simulink model "wbs_sim"  (R2025a)
settings: Solver=FixedStepAuto  StartTime=0.0  StopTime=20  FixedStep=0.001  RelTol=1e-3
undefined symbols (not defined in the file): dyaw, L_l, L_r, phi_1l, phi_1r, phi_4l, phi_4r, roll, theta_l, theta_r, x, X, Y, yaw, Z
libraries: sm_lib x86, nesl_utility x28, slpidlib x6
(part 3 of 4)

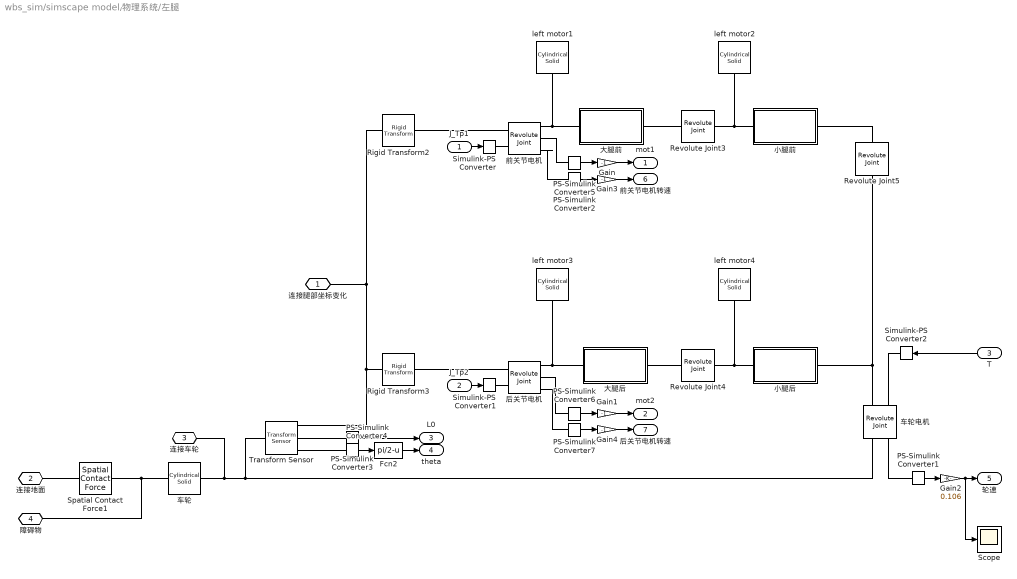
== system wbs_sim/simscape model/物理系统/左腿 ==
  J_Tp1 : Inport
  J_Tp2 : Inport  Port=2
  T : Inport  Port=3
  Fcn2 : Fcn  Expr=pi/2-u
  Gain{,1,3..4} (4 alike) : Gain  Gain=-1
  Gain2 : Gain  Gain=0.106
  PS-Simulink Converter{1..7} (7 alike) : nesl_utility/PS-Simulink Converter  PhysicalDomain=network_engine_domain  SubClassName=ps_output  LeftPortType=input  RightPortType=output  PseudoPeriodic=off  Frequencies=[]  VectorFormat=inherit  Unit=inherit  AffineConversion=off
  Revolute Joint3 : sm_lib/Joints/Revolute Joint  JointMode=Normal  CompositeWrenchDir=FollowerOnBase  CompositeWrenchFrame=BaseFrame  SenseConstraintForce=off  SenseConstraintTorque=off  SenseTotalForce=off  SenseTotalTorque=off  PositionTargetSpecify=on  PositionTargetPriority=Low  PositionTargetValue=-135  PositionTargetValueUnits=deg  VelocityTargetSpecify=off  VelocityTargetPriority=High  VelocityTargetValue=90  VelocityTargetValueUnits=deg/s  EquilibriumPosition=0  EquilibriumPositionUnits=deg  SpringStiffness=0  SpringStiffnessUnits=N*m/deg  DampingCoefficient=0  DampingCoefficientUnits=N*m/(deg/s)  LowerLimitSpecify=off  LowerLimitBound=-90  LowerLimitBoundUnits=deg  LowerLimitStiffness=1e4  LowerLimitStiffnessUnits=N*m/deg  LowerLimitDamping=10  LowerLimitDampingUnits=N*m/(deg/s)  LowerLimitTransitionRegionWidth=0.1  LowerLimitTransitionRegionWidthUnits=deg  UpperLimitSpecify=off  UpperLimitBound=90  UpperLimitBoundUnits=deg  UpperLimitStiffness=1e4  UpperLimitStiffnessUnits=N*m/deg  UpperLimitDamping=10  UpperLimitDampingUnits=N*m/(deg/s)  UpperLimitTransitionRegionWidth=0.1  UpperLimitTransitionRegionWidthUnits=deg  TorqueActuationMode=NoTorque  MotionActuationMode=ComputedMotion  SensePosition=off  SenseVelocity=off  SenseAcceleration=off  SenseTorqueForce=off  SenseLowerLimitTorqueForce=off  SenseUpperLimitTorqueForce=off
  Revolute Joint4 : sm_lib/Joints/Revolute Joint  JointMode=Normal  CompositeWrenchDir=FollowerOnBase  CompositeWrenchFrame=BaseFrame  SenseConstraintForce=off  SenseConstraintTorque=off  SenseTotalForce=off  SenseTotalTorque=off  PositionTargetSpecify=off  PositionTargetPriority=High  PositionTargetValue=0  PositionTargetValueUnits=deg  VelocityTargetSpecify=off  VelocityTargetPriority=High  VelocityTargetValue=90  VelocityTargetValueUnits=deg/s  EquilibriumPosition=0  EquilibriumPositionUnits=deg  SpringStiffness=0  SpringStiffnessUnits=N*m/deg  DampingCoefficient=0  DampingCoefficientUnits=N*m/(deg/s)  LowerLimitSpecify=off  LowerLimitBound=-90  LowerLimitBoundUnits=deg  LowerLimitStiffness=1e4  LowerLimitStiffnessUnits=N*m/deg  LowerLimitDamping=10  LowerLimitDampingUnits=N*m/(deg/s)  LowerLimitTransitionRegionWidth=0.1  LowerLimitTransitionRegionWidthUnits=deg  UpperLimitSpecify=off  UpperLimitBound=90  UpperLimitBoundUnits=deg  UpperLimitStiffness=1e4  UpperLimitStiffnessUnits=N*m/deg  UpperLimitDamping=10  UpperLimitDampingUnits=N*m/(deg/s)  UpperLimitTransitionRegionWidth=0.1  UpperLimitTransitionRegionWidthUnits=deg  TorqueActuationMode=NoTorque  MotionActuationMode=ComputedMotion  SensePosition=off  SenseVelocity=off  SenseAcceleration=off  SenseTorqueForce=off  SenseLowerLimitTorqueForce=off  SenseUpperLimitTorqueForce=off
  Revolute Joint5 : sm_lib/Joints/Revolute Joint  JointMode=Normal  CompositeWrenchDir=FollowerOnBase  CompositeWrenchFrame=BaseFrame  SenseConstraintForce=off  SenseConstraintTorque=off  SenseTotalForce=off  SenseTotalTorque=off  PositionTargetSpecify=off  PositionTargetPriority=High  PositionTargetValue=0  PositionTargetValueUnits=deg  VelocityTargetSpecify=off  VelocityTargetPriority=High  VelocityTargetValue=90  VelocityTargetValueUnits=deg/s  EquilibriumPosition=0  EquilibriumPositionUnits=deg  SpringStiffness=0  SpringStiffnessUnits=N*m/deg  DampingCoefficient=0  DampingCoefficientUnits=N*m/(deg/s)  LowerLimitSpecify=off  LowerLimitBound=-90  LowerLimitBoundUnits=deg  LowerLimitStiffness=1e4  LowerLimitStiffnessUnits=N*m/deg  LowerLimitDamping=10  LowerLimitDampingUnits=N*m/(deg/s)  LowerLimitTransitionRegionWidth=0.1  LowerLimitTransitionRegionWidthUnits=deg  UpperLimitSpecify=off  UpperLimitBound=90  UpperLimitBoundUnits=deg  UpperLimitStiffness=1e4  UpperLimitStiffnessUnits=N*m/deg  UpperLimitDamping=10  UpperLimitDampingUnits=N*m/(deg/s)  UpperLimitTransitionRegionWidth=0.1  UpperLimitTransitionRegionWidthUnits=deg  TorqueActuationMode=NoTorque  MotionActuationMode=ComputedMotion  SensePosition=off  SenseVelocity=off  SenseAcceleration=off  SenseTorqueForce=off  SenseLowerLimitTorqueForce=off  SenseUpperLimitTorqueForce=off
  Rigid Transform2 : sm_lib/Frames and Transforms/Rigid Transform  RotationMethod=None  FollAlignAxisA=+X  BaseAlignAxisA=+Y  FollAlignAxisB=+Y  BaseAlignAxisB=+Z  RotationStandardAxis=+Z  RotationAngle=0.0  RotationAngleUnits=deg  RotationArbitraryAxis=[0 0 1]  RotationSequenceAxes=FollowerAxes  RotationSequence=XYX  RotationSequenceAngles=[0 0 0]  RotationSequenceAnglesUnits=deg  RotationMatrix=[1 0 0; 0 1 0; 0 0 1]  Quaternion=[1 0 0 0]  TranslationMethod=StandardAxis  TranslationCartesianOffset=[0 0 0]  TranslationCartesianOffsetUnits=m  TranslationStandardAxis=+X  TranslationStandardOffset=0.0425  TranslationStandardOffsetUnits=m  TranslationROffset=0  TranslationROffsetUnits=m  TranslationThetaOffset=0  TranslationThetaOffsetUnits=deg  TranslationZOffset=0  TranslationZOffsetUnits=m
  Rigid Transform3 : sm_lib/Frames and Transforms/Rigid Transform  RotationMethod=None  FollAlignAxisA=+X  BaseAlignAxisA=+Y  FollAlignAxisB=+Y  BaseAlignAxisB=+Z  RotationStandardAxis=+Z  RotationAngle=0.0  RotationAngleUnits=deg  RotationArbitraryAxis=[0 0 1]  RotationSequenceAxes=FollowerAxes  RotationSequence=XYX  RotationSequenceAngles=[0 0 0]  RotationSequenceAnglesUnits=deg  RotationMatrix=[1 0 0; 0 1 0; 0 0 1]  Quaternion=[1 0 0 0]  TranslationMethod=StandardAxis  TranslationCartesianOffset=[0 0 0]  TranslationCartesianOffsetUnits=m  TranslationStandardAxis=-X  TranslationStandardOffset=0.0425  TranslationStandardOffsetUnits=m  TranslationROffset=0  TranslationROffsetUnits=m  TranslationThetaOffset=0  TranslationThetaOffsetUnits=deg  TranslationZOffset=0  TranslationZOffsetUnits=m
  Scope : Scope
      settings: ActiveDisplayYMinimum=-32.212491116980587  ActiveDisplayYMaximum=60.605287499899276  DataLoggingVariableName=ScopeData7
  Simulink-PS Converter : nesl_utility/Simulink-PS Converter  PhysicalDomain=network_engine_domain  SubClassName=ps_input  LeftPortType=input  RightPortType=output  PseudoPeriodic=off  Frequencies=[]  NoiseDistribution=none  NoiseParameters=[]  Unit=1  AffineConversion=off  FilteringAndDerivatives=provide  SimscapeFilterOrder=1  InputFilterTimeConstant=0.001  UdotUserProvided=0
  Simulink-PS Converter1 : nesl_utility/Simulink-PS Converter  PhysicalDomain=network_engine_domain  SubClassName=ps_input  LeftPortType=input  RightPortType=output  PseudoPeriodic=off  Frequencies=[]  NoiseDistribution=none  NoiseParameters=[]  Unit=1  AffineConversion=off  FilteringAndDerivatives=provide  SimscapeFilterOrder=1  InputFilterTimeConstant=0.001  UdotUserProvided=0
  Simulink-PS Converter2 : nesl_utility/Simulink-PS Converter  PhysicalDomain=network_engine_domain  SubClassName=ps_input  LeftPortType=input  RightPortType=output  PseudoPeriodic=off  Frequencies=[]  NoiseDistribution=none  NoiseParameters=[]  Unit=1  AffineConversion=off  FilteringAndDerivatives=provide  SimscapeFilterOrder=1  InputFilterTimeConstant=0.001  UdotUserProvided=0
  Spatial Contact Force1 : sm_lib/Forces and Torques/Spatial Contact Force  SenseSeparationDistance=off  NormalForceType=SmoothSpringDamper  NormalStiffness=1e6  NormalStiffnessUnits=N/m  NormalDamping=1e3  NormalDampingUnits=N/(m/s)  NormalTransitionRegionWidth=1e-4  NormalTransitionRegionWidthUnits=m  FrictionType=SmoothStickSlip  CoefficientOfStaticFriction=0.5  CoefficientOfDynamicFriction=0.3  FrictionalCriticalVelocity=1e-3  FrictionalCriticalVelocityUnits=m/s  SenseContactSignal=off  SensePenetrationDepth=off  SenseNormalVelocity=off  SenseTangentialVelocity=off  SensingForceTorqueDirection=BaseOnFollower  SensingForceTorqueResolutionFrame=ContactFrame  SenseNormalForce=off  SenseNormalForceMagnitude=off  SenseNormalTorque=off  SenseFrictionalForce=off  SenseFrictionalForceMagnitude=off  SenseFrictionalTorque=off  SenseTotalForce=off  SenseTotalTorque=off  SenseContactBaseRotation=off  SenseContactBaseTranslation=off  SenseContactFollowerRotation=off  SenseContactFollowerTranslation=off  ZeroCrossDetectContactStartAndEnd=off
  Transform Sensor : sm_lib/Frames and Transforms/Transform Sensor  MeasurementFrame=World  RotationSequence=XYX  SenseAngle=off  SenseAxis=off  SenseQ=off  SenseR=off  SenseRotationSequence=off  SenseOmegaX=off  SenseOmegaY=off  SenseOmegaZ=off  SenseOmega=off  SenseQDot=off  SenseRDot=off  SenseRotationSequenceDot=off  SenseAlphaX=off  SenseAlphaY=off  SenseAlphaZ=off  SenseAlpha=off  SenseQDDot=off  SenseRDDot=off  SenseX=off  SenseY=off  SenseZ=off  SenseXYZ=off  SenseRad=on  SenseAzim=on  SenseDist=off  SenseInc=off  SenseXDot=off  SenseYDot=off  SenseZDot=off  SenseXYZDot=off  SenseRadDot=off  SenseAzimDot=off  SenseDistDot=off  SenseIncDot=off  SenseXDDot=off  SenseYDDot=off  SenseZDDot=off  SenseXYZDDot=off  SenseRadDDot=off  SenseAzimDDot=off  SenseDistDDot=off  SenseIncDDot=off
  left motor{1..4} (4 alike) : sm_lib/Body Elements/Cylindrical Solid  CylinderRadius=0.03  CylinderRadiusUnits=m  CylinderLength=0.02  CylinderLengthUnits=m  ExportEntireGeometry=off  InertiaType=CalculateFromGeometry  BasedOnType=Mass  Density=1000  DensityUnits=kg/m^3  Mass=0  MassUnits=kg  CenterOfMass=[0 0 0]  CenterOfMassUnits=m  MomentsOfInertia=[1 1 1]  MomentsOfInertiaUnits=kg*m^2  ProductsOfInertia=[0 0 0]  ProductsOfInertiaUnits=kg*m^2  GraphicType=FromGeometry  MarkerShape=Sphere  MarkerSize=10  GraphicVisPropType=SimpleVisualProperties  GraphicDiffuseColor=[0.1569 0.1569 0.03137]  GraphicOpacity=1.0  GraphicSpecularColor=[0.5 0.5 0.5 1.0]  GraphicAmbientColor=[0.15 0.15 0.15 1.0]  GraphicEmissiveColor=[0.0 0.0 0.0 1.0]  GraphicShininess=75  DoExposeReferenceFrame=on  SerializedFrames=<Frames/>
  前关节电机 : sm_lib/Joints/Revolute Joint  JointMode=Normal  CompositeWrenchDir=FollowerOnBase  CompositeWrenchFrame=BaseFrame  SenseConstraintForce=off  SenseConstraintTorque=off  SenseTotalForce=off  SenseTotalTorque=off  PositionTargetSpecify=on  PositionTargetPriority=High  PositionTargetValue=-30  PositionTargetValueUnits=deg  VelocityTargetSpecify=off  VelocityTargetPriority=High  VelocityTargetValue=90  VelocityTargetValueUnits=deg/s  EquilibriumPosition=0  EquilibriumPositionUnits=deg  SpringStiffness=0  SpringStiffnessUnits=N*m/deg  DampingCoefficient=0  DampingCoefficientUnits=N*m/(deg/s)  LowerLimitSpecify=off  LowerLimitBound=-90  LowerLimitBoundUnits=deg  LowerLimitStiffness=1e4  LowerLimitStiffnessUnits=N*m/deg  LowerLimitDamping=10  LowerLimitDampingUnits=N*m/(deg/s)  LowerLimitTransitionRegionWidth=0.1  LowerLimitTransitionRegionWidthUnits=deg  UpperLimitSpecify=off  UpperLimitBound=90  UpperLimitBoundUnits=deg  UpperLimitStiffness=1e4  UpperLimitStiffnessUnits=N*m/deg  UpperLimitDamping=10  UpperLimitDampingUnits=N*m/(deg/s)  UpperLimitTransitionRegionWidth=0.1  UpperLimitTransitionRegionWidthUnits=deg  TorqueActuationMode=InputTorque  MotionActuationMode=ComputedMotion  SensePosition=on  SenseVelocity=on  SenseAcceleration=off  SenseTorqueForce=off  SenseLowerLimitTorqueForce=off  SenseUpperLimitTorqueForce=off
  后关节电机 : sm_lib/Joints/Revolute Joint  JointMode=Normal  CompositeWrenchDir=FollowerOnBase  CompositeWrenchFrame=BaseFrame  SenseConstraintForce=off  SenseConstraintTorque=off  SenseTotalForce=off  SenseTotalTorque=off  PositionTargetSpecify=on  PositionTargetPriority=High  PositionTargetValue=210  PositionTargetValueUnits=deg  VelocityTargetSpecify=off  VelocityTargetPriority=High  VelocityTargetValue=90  VelocityTargetValueUnits=deg/s  EquilibriumPosition=0  EquilibriumPositionUnits=deg  SpringStiffness=0  SpringStiffnessUnits=N*m/deg  DampingCoefficient=0  DampingCoefficientUnits=N*m/(deg/s)  LowerLimitSpecify=off  LowerLimitBound=-90  LowerLimitBoundUnits=deg  LowerLimitStiffness=1e4  LowerLimitStiffnessUnits=N*m/deg  LowerLimitDamping=10  LowerLimitDampingUnits=N*m/(deg/s)  LowerLimitTransitionRegionWidth=0.1  LowerLimitTransitionRegionWidthUnits=deg  UpperLimitSpecify=off  UpperLimitBound=90  UpperLimitBoundUnits=deg  UpperLimitStiffness=1e4  UpperLimitStiffnessUnits=N*m/deg  UpperLimitDamping=10  UpperLimitDampingUnits=N*m/(deg/s)  UpperLimitTransitionRegionWidth=0.1  UpperLimitTransitionRegionWidthUnits=deg  TorqueActuationMode=InputTorque  MotionActuationMode=ComputedMotion  SensePosition=on  SenseVelocity=on  SenseAcceleration=off  SenseTorqueForce=off  SenseLowerLimitTorqueForce=off  SenseUpperLimitTorqueForce=off
  大腿前 : Subsystem  mask{L=0.21, W=0.01, H=0.05, mass=0.75}
      mask prompts: L "Length"; W "Width"; H "Height"
  大腿后 : Subsystem  mask{L=0.21, W=0.01, H=0.05, mass=0.75}
      mask prompts: L "Length"; W "Width"; H "Height"
  小腿前 : Subsystem  mask{L=0.25, W=0.01, H=0.05, mass=0.5}
      mask prompts: L "Length"; W "Width"; H "Height"
  小腿后 : Subsystem  mask{L=0.25, W=0.01, H=0.05, mass=0.5}
      mask prompts: L "Length"; W "Width"; H "Height"
  车轮 : sm_lib/Body Elements/Cylindrical Solid  CylinderRadius=0.06  CylinderRadiusUnits=m  CylinderLength=0.03  CylinderLengthUnits=m  ExportEntireGeometry=on  InertiaType=CalculateFromGeometry  BasedOnType=Mass  Density=661  DensityUnits=kg/m^3  Mass=0.5  MassUnits=kg  CenterOfMass=[0 0 0]  CenterOfMassUnits=m  MomentsOfInertia=[1 1 1]  MomentsOfInertiaUnits=kg*m^2  ProductsOfInertia=[0 0 0]  ProductsOfInertiaUnits=kg*m^2  GraphicType=FromGeometry  MarkerShape=Sphere  MarkerSize=10  GraphicVisPropType=SimpleVisualProperties  GraphicDiffuseColor=[1 0 0]  GraphicOpacity=1.0  GraphicSpecularColor=[0.5 0.5 0.5 1.0]  GraphicAmbientColor=[0.15 0.15 0.15 1.0]  GraphicEmissiveColor=[0.0 0.0 0.0 1.0]  GraphicShininess=75  DoExposeReferenceFrame=on  SerializedFrames=<Frames/>
  车轮电机 : sm_lib/Joints/Revolute Joint  JointMode=Normal  CompositeWrenchDir=FollowerOnBase  CompositeWrenchFrame=BaseFrame  SenseConstraintForce=off  SenseConstraintTorque=off  SenseTotalForce=off  SenseTotalTorque=off  PositionTargetSpecify=off  PositionTargetPriority=High  PositionTargetValue=0  PositionTargetValueUnits=deg  VelocityTargetSpecify=off  VelocityTargetPriority=High  VelocityTargetValue=90  VelocityTargetValueUnits=deg/s  EquilibriumPosition=0  EquilibriumPositionUnits=deg  SpringStiffness=0  SpringStiffnessUnits=N*m/deg  DampingCoefficient=0  DampingCoefficientUnits=N*m/(deg/s)  LowerLimitSpecify=off  LowerLimitBound=-90  LowerLimitBoundUnits=deg  LowerLimitStiffness=1e4  LowerLimitStiffnessUnits=N*m/deg  LowerLimitDamping=10  LowerLimitDampingUnits=N*m/(deg/s)  LowerLimitTransitionRegionWidth=0.1  LowerLimitTransitionRegionWidthUnits=deg  UpperLimitSpecify=off  UpperLimitBound=90  UpperLimitBoundUnits=deg  UpperLimitStiffness=1e4  UpperLimitStiffnessUnits=N*m/deg  UpperLimitDamping=10  UpperLimitDampingUnits=N*m/(deg/s)  UpperLimitTransitionRegionWidth=0.1  UpperLimitTransitionRegionWidthUnits=deg  TorqueActuationMode=InputTorque  MotionActuationMode=ComputedMotion  SensePosition=off  SenseVelocity=on  SenseAcceleration=off  SenseTorqueForce=off  SenseLowerLimitTorqueForce=off  SenseUpperLimitTorqueForce=off
  连接腿部坐标变化 : PMIOPort  Side=Left
  连接地面 : PMIOPort  Port=2  Side=Left
  连接车轮 : PMIOPort  Port=3  Side=Left
  障碍物 : PMIOPort  Port=4  Side=Left
  mot1 : Outport
  mot2 : Outport  Port=2
  L0 : Outport  Port=3
  theta : Outport  Port=4
  轮速 : Outport  Port=5
  前关节电机转速 : Outport  Port=6
  后关节电机转速 : Outport  Port=7
  wires:
  T/1 -> Simulink-PS Converter2/1
  J_Tp2/1 -> Simulink-PS Converter1/1
  J_Tp1/1 -> Simulink-PS Converter/1
  Gain/1 -> mot1/1
  PS-Simulink Converter5/1 -> Gain/1
  Gain1/1 -> mot2/1
  PS-Simulink Converter6/1 -> Gain1/1
  PS-Simulink Converter3/1 -> L0/1
  Fcn2/1 -> theta/1
  PS-Simulink Converter4/1 -> Fcn2/1
  Gain2/1 -> Scope/1, 轮速/1
  PS-Simulink Converter1/1 -> Gain2/1
  PS-Simulink Converter2/1 -> Gain3/1
  Gain3/1 -> 前关节电机转速/1
  Gain4/1 -> 后关节电机转速/1
  PS-Simulink Converter7/1 -> Gain4/1
  connections:
  前关节电机/LConn1 -- Rigid Transform2/RConn1
  Simulink-PS Converter1/RConn1 -- 后关节电机/LConn2
  Simulink-PS Converter2/RConn1 -- 车轮电机/LConn2
  Rigid Transform2/LConn1 -- Transform Sensor/RConn1 -- Rigid Transform3/LConn1 -- 连接腿部坐标变化/RConn1
  车轮电机/LConn1 -- 小腿后/RConn1 -- Revolute Joint5/LConn1
  Revolute Joint4/LConn1 -- 大腿后/RConn1
  车轮/LConn1 -- 障碍物/RConn1 -- Spatial Contact Force1/RConn1
  大腿后/LConn1 -- left motor3/RConn1 -- 后关节电机/RConn1
  后关节电机/LConn1 -- Rigid Transform3/RConn1
  Simulink-PS Converter/RConn1 -- 前关节电机/LConn2
  大腿前/LConn1 -- left motor1/RConn1 -- 前关节电机/RConn1
  Revolute Joint3/LConn1 -- 大腿前/RConn1
  小腿后/LConn1 -- left motor4/RConn1 -- Revolute Joint4/RConn1
  Revolute Joint3/RConn1 -- left motor2/RConn1 -- 小腿前/LConn1
  车轮/RConn1 -- 车轮电机/RConn1 -- Transform Sensor/LConn1 -- 连接车轮/RConn1
  小腿前/RConn1 -- Revolute Joint5/RConn1
  Spatial Contact Force1/LConn1 -- 连接地面/RConn1
  PS-Simulink Converter5/LConn1 -- 前关节电机/RConn2
  后关节电机/RConn2 -- PS-Simulink Converter6/LConn1
  PS-Simulink Converter3/LConn1 -- Transform Sensor/RConn2
  Transform Sensor/RConn3 -- PS-Simulink Converter4/LConn1
  PS-Simulink Converter1/LConn1 -- 车轮电机/RConn2
  前关节电机/RConn3 -- PS-Simulink Converter2/LConn1
  后关节电机/RConn3 -- PS-Simulink Converter7/LConn1

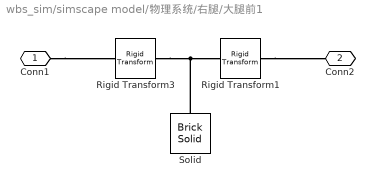
== system wbs_sim/simscape model/物理系统/右腿/大腿前1 ==
  Rigid Transform1 : sm_lib/Frames and Transforms/Rigid Transform  RotationMethod=None  FollAlignAxisA=+X  BaseAlignAxisA=+Y  FollAlignAxisB=+Y  BaseAlignAxisB=+Z  RotationStandardAxis=+Z  RotationAngle=0.0  RotationAngleUnits=deg  RotationArbitraryAxis=[0 0 1]  RotationSequenceAxes=FollowerAxes  RotationSequence=XYX  RotationSequenceAngles=[0 0 0]  RotationSequenceAnglesUnits=deg  RotationMatrix=[1 0 0; 0 1 0; 0 0 1]  Quaternion=[1 0 0 0]  TranslationMethod=StandardAxis  TranslationCartesianOffset=[0 0 0]  TranslationCartesianOffsetUnits=m  TranslationStandardAxis=+X  TranslationStandardOffset=L/2  TranslationStandardOffsetUnits=m  TranslationROffset=0  TranslationROffsetUnits=m  TranslationThetaOffset=0  TranslationThetaOffsetUnits=deg  TranslationZOffset=0  TranslationZOffsetUnits=m
  Rigid Transform3 : sm_lib/Frames and Transforms/Rigid Transform  RotationMethod=None  FollAlignAxisA=+X  BaseAlignAxisA=+Y  FollAlignAxisB=+Y  BaseAlignAxisB=+Z  RotationStandardAxis=+Z  RotationAngle=0.0  RotationAngleUnits=deg  RotationArbitraryAxis=[0 0 1]  RotationSequenceAxes=FollowerAxes  RotationSequence=XYX  RotationSequenceAngles=[0 0 0]  RotationSequenceAnglesUnits=deg  RotationMatrix=[1 0 0; 0 1 0; 0 0 1]  Quaternion=[1 0 0 0]  TranslationMethod=StandardAxis  TranslationCartesianOffset=[0 0 0]  TranslationCartesianOffsetUnits=m  TranslationStandardAxis=+X  TranslationStandardOffset=L/2  TranslationStandardOffsetUnits=m  TranslationROffset=0  TranslationROffsetUnits=m  TranslationThetaOffset=0  TranslationThetaOffsetUnits=deg  TranslationZOffset=0  TranslationZOffsetUnits=m
  Solid : sm_lib/Body Elements/Brick Solid  BrickDimensions=[L H W]  BrickDimensionsUnits=m  ExportEntireGeometry=off  InertiaType=CalculateFromGeometry  BasedOnType=Mass  Density=Mass  DensityUnits=kg/m^3  Mass=mass  MassUnits=kg  CenterOfMass=[0 0 0]  CenterOfMassUnits=m  MomentsOfInertia=[1 1 1]  MomentsOfInertiaUnits=kg*m^2  ProductsOfInertia=[0 0 0]  ProductsOfInertiaUnits=kg*m^2  GraphicType=FromGeometry  MarkerShape=Sphere  MarkerSize=10  GraphicVisPropType=SimpleVisualProperties  GraphicDiffuseColor=[0.6667 0 1]  GraphicOpacity=1.0  GraphicSpecularColor=[0.5 0.5 0.5 1.0]  GraphicAmbientColor=[0.15 0.15 0.15 1.0]  GraphicEmissiveColor=[0.0 0.0 0.0 1.0]  GraphicShininess=75  DoExposeReferenceFrame=on  SerializedFrames=<Frames/>
  Conn1 : PMIOPort  Side=Left
  Conn2 : PMIOPort  Port=2  Side=Right
  connections:
  Solid/RConn1 -- Rigid Transform3/RConn1 -- Rigid Transform1/LConn1
  Conn1/RConn1 -- Rigid Transform3/LConn1
  Rigid Transform1/RConn1 -- Conn2/RConn1

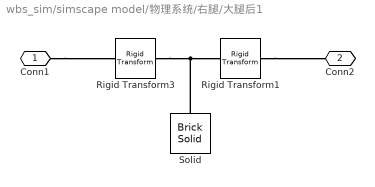
== system wbs_sim/simscape model/物理系统/右腿/大腿后1 ==
  Rigid Transform1 : sm_lib/Frames and Transforms/Rigid Transform  RotationMethod=None  FollAlignAxisA=+X  BaseAlignAxisA=+Y  FollAlignAxisB=+Y  BaseAlignAxisB=+Z  RotationStandardAxis=+Z  RotationAngle=0.0  RotationAngleUnits=deg  RotationArbitraryAxis=[0 0 1]  RotationSequenceAxes=FollowerAxes  RotationSequence=XYX  RotationSequenceAngles=[0 0 0]  RotationSequenceAnglesUnits=deg  RotationMatrix=[1 0 0; 0 1 0; 0 0 1]  Quaternion=[1 0 0 0]  TranslationMethod=StandardAxis  TranslationCartesianOffset=[0 0 0]  TranslationCartesianOffsetUnits=m  TranslationStandardAxis=+X  TranslationStandardOffset=L/2  TranslationStandardOffsetUnits=m  TranslationROffset=0  TranslationROffsetUnits=m  TranslationThetaOffset=0  TranslationThetaOffsetUnits=deg  TranslationZOffset=0  TranslationZOffsetUnits=m
  Rigid Transform3 : sm_lib/Frames and Transforms/Rigid Transform  RotationMethod=None  FollAlignAxisA=+X  BaseAlignAxisA=+Y  FollAlignAxisB=+Y  BaseAlignAxisB=+Z  RotationStandardAxis=+Z  RotationAngle=0.0  RotationAngleUnits=deg  RotationArbitraryAxis=[0 0 1]  RotationSequenceAxes=FollowerAxes  RotationSequence=XYX  RotationSequenceAngles=[0 0 0]  RotationSequenceAnglesUnits=deg  RotationMatrix=[1 0 0; 0 1 0; 0 0 1]  Quaternion=[1 0 0 0]  TranslationMethod=StandardAxis  TranslationCartesianOffset=[0 0 0]  TranslationCartesianOffsetUnits=m  TranslationStandardAxis=+X  TranslationStandardOffset=L/2  TranslationStandardOffsetUnits=m  TranslationROffset=0  TranslationROffsetUnits=m  TranslationThetaOffset=0  TranslationThetaOffsetUnits=deg  TranslationZOffset=0  TranslationZOffsetUnits=m
  Solid : sm_lib/Body Elements/Brick Solid  BrickDimensions=[L H W]  BrickDimensionsUnits=m  ExportEntireGeometry=off  InertiaType=CalculateFromGeometry  BasedOnType=Mass  Density=Mass  DensityUnits=kg/m^3  Mass=mass  MassUnits=kg  CenterOfMass=[0 0 0]  CenterOfMassUnits=m  MomentsOfInertia=[1 1 1]  MomentsOfInertiaUnits=kg*m^2  ProductsOfInertia=[0 0 0]  ProductsOfInertiaUnits=kg*m^2  GraphicType=FromGeometry  MarkerShape=Sphere  MarkerSize=10  GraphicVisPropType=SimpleVisualProperties  GraphicDiffuseColor=[0.6667 0 1]  GraphicOpacity=1.0  GraphicSpecularColor=[0.5 0.5 0.5 1.0]  GraphicAmbientColor=[0.15 0.15 0.15 1.0]  GraphicEmissiveColor=[0.0 0.0 0.0 1.0]  GraphicShininess=75  DoExposeReferenceFrame=on  SerializedFrames=<Frames/>
  Conn1 : PMIOPort  Side=Left
  Conn2 : PMIOPort  Port=2  Side=Right
  connections:
  Solid/RConn1 -- Rigid Transform3/RConn1 -- Rigid Transform1/LConn1
  Conn1/RConn1 -- Rigid Transform3/LConn1
  Rigid Transform1/RConn1 -- Conn2/RConn1

== system wbs_sim/simscape model/物理系统/右腿/小腿前1 ==
  Rigid Transform1 : sm_lib/Frames and Transforms/Rigid Transform  RotationMethod=None  FollAlignAxisA=+X  BaseAlignAxisA=+Y  FollAlignAxisB=+Y  BaseAlignAxisB=+Z  RotationStandardAxis=+Z  RotationAngle=0.0  RotationAngleUnits=deg  RotationArbitraryAxis=[0 0 1]  RotationSequenceAxes=FollowerAxes  RotationSequence=XYX  RotationSequenceAngles=[0 0 0]  RotationSequenceAnglesUnits=deg  RotationMatrix=[1 0 0; 0 1 0; 0 0 1]  Quaternion=[1 0 0 0]  TranslationMethod=StandardAxis  TranslationCartesianOffset=[0 0 0]  TranslationCartesianOffsetUnits=m  TranslationStandardAxis=+X  TranslationStandardOffset=L/2  TranslationStandardOffsetUnits=m  TranslationROffset=0  TranslationROffsetUnits=m  TranslationThetaOffset=0  TranslationThetaOffsetUnits=deg  TranslationZOffset=0  TranslationZOffsetUnits=m
  Rigid Transform3 : sm_lib/Frames and Transforms/Rigid Transform  RotationMethod=None  FollAlignAxisA=+X  BaseAlignAxisA=+Y  FollAlignAxisB=+Y  BaseAlignAxisB=+Z  RotationStandardAxis=+Z  RotationAngle=0.0  RotationAngleUnits=deg  RotationArbitraryAxis=[0 0 1]  RotationSequenceAxes=FollowerAxes  RotationSequence=XYX  RotationSequenceAngles=[0 0 0]  RotationSequenceAnglesUnits=deg  RotationMatrix=[1 0 0; 0 1 0; 0 0 1]  Quaternion=[1 0 0 0]  TranslationMethod=StandardAxis  TranslationCartesianOffset=[0 0 0]  TranslationCartesianOffsetUnits=m  TranslationStandardAxis=+X  TranslationStandardOffset=L/2  TranslationStandardOffsetUnits=m  TranslationROffset=0  TranslationROffsetUnits=m  TranslationThetaOffset=0  TranslationThetaOffsetUnits=deg  TranslationZOffset=0  TranslationZOffsetUnits=m
  Solid : sm_lib/Body Elements/Brick Solid  BrickDimensions=[L H W]  BrickDimensionsUnits=m  ExportEntireGeometry=off  InertiaType=CalculateFromGeometry  BasedOnType=Mass  Density=mass  DensityUnits=kg/m^3  Mass=mass  MassUnits=kg  CenterOfMass=[0 0 0]  CenterOfMassUnits=m  MomentsOfInertia=[1 1 1]  MomentsOfInertiaUnits=kg*m^2  ProductsOfInertia=[0 0 0]  ProductsOfInertiaUnits=kg*m^2  GraphicType=FromGeometry  MarkerShape=Sphere  MarkerSize=10  GraphicVisPropType=SimpleVisualProperties  GraphicDiffuseColor=[1 0 1]  GraphicOpacity=1.0  GraphicSpecularColor=[0.5 0.5 0.5 1.0]  GraphicAmbientColor=[0.15 0.15 0.15 1.0]  GraphicEmissiveColor=[0.0 0.0 0.0 1.0]  GraphicShininess=75  DoExposeReferenceFrame=on  SerializedFrames=<Frames/>
  Conn1 : PMIOPort  Side=Left
  Conn2 : PMIOPort  Port=2  Side=Right
  connections:
  Rigid Transform1/RConn1 -- Conn2/RConn1
  Conn1/RConn1 -- Rigid Transform3/LConn1
  Rigid Transform1/LConn1 -- Solid/RConn1 -- Rigid Transform3/RConn1

== system wbs_sim/simscape model/物理系统/右腿/小腿后1 ==
  Rigid Transform1 : sm_lib/Frames and Transforms/Rigid Transform  RotationMethod=None  FollAlignAxisA=+X  BaseAlignAxisA=+Y  FollAlignAxisB=+Y  BaseAlignAxisB=+Z  RotationStandardAxis=+Z  RotationAngle=0.0  RotationAngleUnits=deg  RotationArbitraryAxis=[0 0 1]  RotationSequenceAxes=FollowerAxes  RotationSequence=XYX  RotationSequenceAngles=[0 0 0]  RotationSequenceAnglesUnits=deg  RotationMatrix=[1 0 0; 0 1 0; 0 0 1]  Quaternion=[1 0 0 0]  TranslationMethod=StandardAxis  TranslationCartesianOffset=[0 0 0]  TranslationCartesianOffsetUnits=m  TranslationStandardAxis=+X  TranslationStandardOffset=L/2  TranslationStandardOffsetUnits=m  TranslationROffset=0  TranslationROffsetUnits=m  TranslationThetaOffset=0  TranslationThetaOffsetUnits=deg  TranslationZOffset=0  TranslationZOffsetUnits=m
  Rigid Transform3 : sm_lib/Frames and Transforms/Rigid Transform  RotationMethod=None  FollAlignAxisA=+X  BaseAlignAxisA=+Y  FollAlignAxisB=+Y  BaseAlignAxisB=+Z  RotationStandardAxis=+Z  RotationAngle=0.0  RotationAngleUnits=deg  RotationArbitraryAxis=[0 0 1]  RotationSequenceAxes=FollowerAxes  RotationSequence=XYX  RotationSequenceAngles=[0 0 0]  RotationSequenceAnglesUnits=deg  RotationMatrix=[1 0 0; 0 1 0; 0 0 1]  Quaternion=[1 0 0 0]  TranslationMethod=StandardAxis  TranslationCartesianOffset=[0 0 0]  TranslationCartesianOffsetUnits=m  TranslationStandardAxis=+X  TranslationStandardOffset=L/2  TranslationStandardOffsetUnits=m  TranslationROffset=0  TranslationROffsetUnits=m  TranslationThetaOffset=0  TranslationThetaOffsetUnits=deg  TranslationZOffset=0  TranslationZOffsetUnits=m
  Solid : sm_lib/Body Elements/Brick Solid  BrickDimensions=[L H W]  BrickDimensionsUnits=m  ExportEntireGeometry=off  InertiaType=CalculateFromGeometry  BasedOnType=Mass  Density=mass  DensityUnits=kg/m^3  Mass=mass  MassUnits=kg  CenterOfMass=[0 0 0]  CenterOfMassUnits=m  MomentsOfInertia=[1 1 1]  MomentsOfInertiaUnits=kg*m^2  ProductsOfInertia=[0 0 0]  ProductsOfInertiaUnits=kg*m^2  GraphicType=FromGeometry  MarkerShape=Sphere  MarkerSize=10  GraphicVisPropType=SimpleVisualProperties  GraphicDiffuseColor=[1 0 1]  GraphicOpacity=1.0  GraphicSpecularColor=[0.5 0.5 0.5 1.0]  GraphicAmbientColor=[0.15 0.15 0.15 1.0]  GraphicEmissiveColor=[0.0 0.0 0.0 1.0]  GraphicShininess=75  DoExposeReferenceFrame=on  SerializedFrames=<Frames/>
  Conn1 : PMIOPort  Side=Left
  Conn2 : PMIOPort  Port=2  Side=Right
  connections:
  Rigid Transform1/RConn1 -- Conn2/RConn1
  Conn1/RConn1 -- Rigid Transform3/LConn1
  Rigid Transform1/LConn1 -- Solid/RConn1 -- Rigid Transform3/RConn1

== system wbs_sim/simscape model/物理系统/左腿/大腿前 ==
  Rigid Transform1 : sm_lib/Frames and Transforms/Rigid Transform  RotationMethod=None  FollAlignAxisA=+X  BaseAlignAxisA=+Y  FollAlignAxisB=+Y  BaseAlignAxisB=+Z  RotationStandardAxis=+Z  RotationAngle=0.0  RotationAngleUnits=deg  RotationArbitraryAxis=[0 0 1]  RotationSequenceAxes=FollowerAxes  RotationSequence=XYX  RotationSequenceAngles=[0 0 0]  RotationSequenceAnglesUnits=deg  RotationMatrix=[1 0 0; 0 1 0; 0 0 1]  Quaternion=[1 0 0 0]  TranslationMethod=StandardAxis  TranslationCartesianOffset=[0 0 0]  TranslationCartesianOffsetUnits=m  TranslationStandardAxis=+X  TranslationStandardOffset=L/2  TranslationStandardOffsetUnits=m  TranslationROffset=0  TranslationROffsetUnits=m  TranslationThetaOffset=0  TranslationThetaOffsetUnits=deg  TranslationZOffset=0  TranslationZOffsetUnits=m
  Rigid Transform3 : sm_lib/Frames and Transforms/Rigid Transform  RotationMethod=None  FollAlignAxisA=+X  BaseAlignAxisA=+Y  FollAlignAxisB=+Y  BaseAlignAxisB=+Z  RotationStandardAxis=+Z  RotationAngle=0.0  RotationAngleUnits=deg  RotationArbitraryAxis=[0 0 1]  RotationSequenceAxes=FollowerAxes  RotationSequence=XYX  RotationSequenceAngles=[0 0 0]  RotationSequenceAnglesUnits=deg  RotationMatrix=[1 0 0; 0 1 0; 0 0 1]  Quaternion=[1 0 0 0]  TranslationMethod=StandardAxis  TranslationCartesianOffset=[0 0 0]  TranslationCartesianOffsetUnits=m  TranslationStandardAxis=+X  TranslationStandardOffset=L/2  TranslationStandardOffsetUnits=m  TranslationROffset=0  TranslationROffsetUnits=m  TranslationThetaOffset=0  TranslationThetaOffsetUnits=deg  TranslationZOffset=0  TranslationZOffsetUnits=m
  Solid : sm_lib/Body Elements/Brick Solid  BrickDimensions=[L H W]  BrickDimensionsUnits=m  ExportEntireGeometry=off  InertiaType=CalculateFromGeometry  BasedOnType=Mass  Density=Mass  DensityUnits=kg/m^3  Mass=mass  MassUnits=kg  CenterOfMass=[0 0 0]  CenterOfMassUnits=m  MomentsOfInertia=[1 1 1]  MomentsOfInertiaUnits=kg*m^2  ProductsOfInertia=[0 0 0]  ProductsOfInertiaUnits=kg*m^2  GraphicType=FromGeometry  MarkerShape=Sphere  MarkerSize=10  GraphicVisPropType=SimpleVisualProperties  GraphicDiffuseColor=[0.6667 0 1]  GraphicOpacity=1.0  GraphicSpecularColor=[0.5 0.5 0.5 1.0]  GraphicAmbientColor=[0.15 0.15 0.15 1.0]  GraphicEmissiveColor=[0.0 0.0 0.0 1.0]  GraphicShininess=75  DoExposeReferenceFrame=on  SerializedFrames=<Frames/>
  Conn1 : PMIOPort  Side=Left
  Conn2 : PMIOPort  Port=2  Side=Right
  connections:
  Solid/RConn1 -- Rigid Transform3/RConn1 -- Rigid Transform1/LConn1
  Conn1/RConn1 -- Rigid Transform3/LConn1
  Rigid Transform1/RConn1 -- Conn2/RConn1

== system wbs_sim/simscape model/物理系统/左腿/大腿后 ==
  Rigid Transform1 : sm_lib/Frames and Transforms/Rigid Transform  RotationMethod=None  FollAlignAxisA=+X  BaseAlignAxisA=+Y  FollAlignAxisB=+Y  BaseAlignAxisB=+Z  RotationStandardAxis=+Z  RotationAngle=0.0  RotationAngleUnits=deg  RotationArbitraryAxis=[0 0 1]  RotationSequenceAxes=FollowerAxes  RotationSequence=XYX  RotationSequenceAngles=[0 0 0]  RotationSequenceAnglesUnits=deg  RotationMatrix=[1 0 0; 0 1 0; 0 0 1]  Quaternion=[1 0 0 0]  TranslationMethod=StandardAxis  TranslationCartesianOffset=[0 0 0]  TranslationCartesianOffsetUnits=m  TranslationStandardAxis=+X  TranslationStandardOffset=L/2  TranslationStandardOffsetUnits=m  TranslationROffset=0  TranslationROffsetUnits=m  TranslationThetaOffset=0  TranslationThetaOffsetUnits=deg  TranslationZOffset=0  TranslationZOffsetUnits=m
  Rigid Transform3 : sm_lib/Frames and Transforms/Rigid Transform  RotationMethod=None  FollAlignAxisA=+X  BaseAlignAxisA=+Y  FollAlignAxisB=+Y  BaseAlignAxisB=+Z  RotationStandardAxis=+Z  RotationAngle=0.0  RotationAngleUnits=deg  RotationArbitraryAxis=[0 0 1]  RotationSequenceAxes=FollowerAxes  RotationSequence=XYX  RotationSequenceAngles=[0 0 0]  RotationSequenceAnglesUnits=deg  RotationMatrix=[1 0 0; 0 1 0; 0 0 1]  Quaternion=[1 0 0 0]  TranslationMethod=StandardAxis  TranslationCartesianOffset=[0 0 0]  TranslationCartesianOffsetUnits=m  TranslationStandardAxis=+X  TranslationStandardOffset=L/2  TranslationStandardOffsetUnits=m  TranslationROffset=0  TranslationROffsetUnits=m  TranslationThetaOffset=0  TranslationThetaOffsetUnits=deg  TranslationZOffset=0  TranslationZOffsetUnits=m
  Solid : sm_lib/Body Elements/Brick Solid  BrickDimensions=[L H W]  BrickDimensionsUnits=m  ExportEntireGeometry=off  InertiaType=CalculateFromGeometry  BasedOnType=Mass  Density=Mass  DensityUnits=kg/m^3  Mass=mass  MassUnits=kg  CenterOfMass=[0 0 0]  CenterOfMassUnits=m  MomentsOfInertia=[1 1 1]  MomentsOfInertiaUnits=kg*m^2  ProductsOfInertia=[0 0 0]  ProductsOfInertiaUnits=kg*m^2  GraphicType=FromGeometry  MarkerShape=Sphere  MarkerSize=10  GraphicVisPropType=SimpleVisualProperties  GraphicDiffuseColor=[0.6667 0 1]  GraphicOpacity=1.0  GraphicSpecularColor=[0.5 0.5 0.5 1.0]  GraphicAmbientColor=[0.15 0.15 0.15 1.0]  GraphicEmissiveColor=[0.0 0.0 0.0 1.0]  GraphicShininess=75  DoExposeReferenceFrame=on  SerializedFrames=<Frames/>
  Conn1 : PMIOPort  Side=Left
  Conn2 : PMIOPort  Port=2  Side=Right
  connections:
  Solid/RConn1 -- Rigid Transform3/RConn1 -- Rigid Transform1/LConn1
  Conn1/RConn1 -- Rigid Transform3/LConn1
  Rigid Transform1/RConn1 -- Conn2/RConn1

== system wbs_sim/simscape model/物理系统/左腿/小腿前 ==
  Rigid Transform1 : sm_lib/Frames and Transforms/Rigid Transform  RotationMethod=None  FollAlignAxisA=+X  BaseAlignAxisA=+Y  FollAlignAxisB=+Y  BaseAlignAxisB=+Z  RotationStandardAxis=+Z  RotationAngle=0.0  RotationAngleUnits=deg  RotationArbitraryAxis=[0 0 1]  RotationSequenceAxes=FollowerAxes  RotationSequence=XYX  RotationSequenceAngles=[0 0 0]  RotationSequenceAnglesUnits=deg  RotationMatrix=[1 0 0; 0 1 0; 0 0 1]  Quaternion=[1 0 0 0]  TranslationMethod=StandardAxis  TranslationCartesianOffset=[0 0 0]  TranslationCartesianOffsetUnits=m  TranslationStandardAxis=+X  TranslationStandardOffset=L/2  TranslationStandardOffsetUnits=m  TranslationROffset=0  TranslationROffsetUnits=m  TranslationThetaOffset=0  TranslationThetaOffsetUnits=deg  TranslationZOffset=0  TranslationZOffsetUnits=m
  Rigid Transform3 : sm_lib/Frames and Transforms/Rigid Transform  RotationMethod=None  FollAlignAxisA=+X  BaseAlignAxisA=+Y  FollAlignAxisB=+Y  BaseAlignAxisB=+Z  RotationStandardAxis=+Z  RotationAngle=0.0  RotationAngleUnits=deg  RotationArbitraryAxis=[0 0 1]  RotationSequenceAxes=FollowerAxes  RotationSequence=XYX  RotationSequenceAngles=[0 0 0]  RotationSequenceAnglesUnits=deg  RotationMatrix=[1 0 0; 0 1 0; 0 0 1]  Quaternion=[1 0 0 0]  TranslationMethod=StandardAxis  TranslationCartesianOffset=[0 0 0]  TranslationCartesianOffsetUnits=m  TranslationStandardAxis=+X  TranslationStandardOffset=L/2  TranslationStandardOffsetUnits=m  TranslationROffset=0  TranslationROffsetUnits=m  TranslationThetaOffset=0  TranslationThetaOffsetUnits=deg  TranslationZOffset=0  TranslationZOffsetUnits=m
  Solid : sm_lib/Body Elements/Brick Solid  BrickDimensions=[L H W]  BrickDimensionsUnits=m  ExportEntireGeometry=off  InertiaType=CalculateFromGeometry  BasedOnType=Mass  Density=mass  DensityUnits=kg/m^3  Mass=mass  MassUnits=kg  CenterOfMass=[0 0 0]  CenterOfMassUnits=m  MomentsOfInertia=[1 1 1]  MomentsOfInertiaUnits=kg*m^2  ProductsOfInertia=[0 0 0]  ProductsOfInertiaUnits=kg*m^2  GraphicType=FromGeometry  MarkerShape=Sphere  MarkerSize=10  GraphicVisPropType=SimpleVisualProperties  GraphicDiffuseColor=[1 0 1]  GraphicOpacity=1.0  GraphicSpecularColor=[0.5 0.5 0.5 1.0]  GraphicAmbientColor=[0.15 0.15 0.15 1.0]  GraphicEmissiveColor=[0.0 0.0 0.0 1.0]  GraphicShininess=75  DoExposeReferenceFrame=on  SerializedFrames=<Frames/>
  Conn1 : PMIOPort  Side=Left
  Conn2 : PMIOPort  Port=2  Side=Right
  connections:
  Rigid Transform1/RConn1 -- Conn2/RConn1
  Conn1/RConn1 -- Rigid Transform3/LConn1
  Rigid Transform1/LConn1 -- Solid/RConn1 -- Rigid Transform3/RConn1

== system wbs_sim/simscape model/物理系统/左腿/小腿后 ==
  Rigid Transform1 : sm_lib/Frames and Transforms/Rigid Transform  RotationMethod=None  FollAlignAxisA=+X  BaseAlignAxisA=+Y  FollAlignAxisB=+Y  BaseAlignAxisB=+Z  RotationStandardAxis=+Z  RotationAngle=0.0  RotationAngleUnits=deg  RotationArbitraryAxis=[0 0 1]  RotationSequenceAxes=FollowerAxes  RotationSequence=XYX  RotationSequenceAngles=[0 0 0]  RotationSequenceAnglesUnits=deg  RotationMatrix=[1 0 0; 0 1 0; 0 0 1]  Quaternion=[1 0 0 0]  TranslationMethod=StandardAxis  TranslationCartesianOffset=[0 0 0]  TranslationCartesianOffsetUnits=m  TranslationStandardAxis=+X  TranslationStandardOffset=L/2  TranslationStandardOffsetUnits=m  TranslationROffset=0  TranslationROffsetUnits=m  TranslationThetaOffset=0  TranslationThetaOffsetUnits=deg  TranslationZOffset=0  TranslationZOffsetUnits=m
  Rigid Transform3 : sm_lib/Frames and Transforms/Rigid Transform  RotationMethod=None  FollAlignAxisA=+X  BaseAlignAxisA=+Y  FollAlignAxisB=+Y  BaseAlignAxisB=+Z  RotationStandardAxis=+Z  RotationAngle=0.0  RotationAngleUnits=deg  RotationArbitraryAxis=[0 0 1]  RotationSequenceAxes=FollowerAxes  RotationSequence=XYX  RotationSequenceAngles=[0 0 0]  RotationSequenceAnglesUnits=deg  RotationMatrix=[1 0 0; 0 1 0; 0 0 1]  Quaternion=[1 0 0 0]  TranslationMethod=StandardAxis  TranslationCartesianOffset=[0 0 0]  TranslationCartesianOffsetUnits=m  TranslationStandardAxis=+X  TranslationStandardOffset=L/2  TranslationStandardOffsetUnits=m  TranslationROffset=0  TranslationROffsetUnits=m  TranslationThetaOffset=0  TranslationThetaOffsetUnits=deg  TranslationZOffset=0  TranslationZOffsetUnits=m
  Solid : sm_lib/Body Elements/Brick Solid  BrickDimensions=[L H W]  BrickDimensionsUnits=m  ExportEntireGeometry=off  InertiaType=CalculateFromGeometry  BasedOnType=Mass  Density=mass  DensityUnits=kg/m^3  Mass=mass  MassUnits=kg  CenterOfMass=[0 0 0]  CenterOfMassUnits=m  MomentsOfInertia=[1 1 1]  MomentsOfInertiaUnits=kg*m^2  ProductsOfInertia=[0 0 0]  ProductsOfInertiaUnits=kg*m^2  GraphicType=FromGeometry  MarkerShape=Sphere  MarkerSize=10  GraphicVisPropType=SimpleVisualProperties  GraphicDiffuseColor=[1 0 1]  GraphicOpacity=1.0  GraphicSpecularColor=[0.5 0.5 0.5 1.0]  GraphicAmbientColor=[0.15 0.15 0.15 1.0]  GraphicEmissiveColor=[0.0 0.0 0.0 1.0]  GraphicShininess=75  DoExposeReferenceFrame=on  SerializedFrames=<Frames/>
  Conn1 : PMIOPort  Side=Left
  Conn2 : PMIOPort  Port=2  Side=Right
  connections:
  Rigid Transform1/RConn1 -- Conn2/RConn1
  Conn1/RConn1 -- Rigid Transform3/LConn1
  Rigid Transform1/LConn1 -- Solid/RConn1 -- Rigid Transform3/RConn1

== matlab function wbs_sim/controller/left leg transform ==
  data: F input; Tp input; T output; phi1 input; phi4 input
function T = LegTransform(F,Tp,phi1,phi4)
%LegTransform
%    T = LegTransform(F,Tp,PHI1,PHI4)

%    This function was generated by the Symbolic Math Toolbox version 25.1.
%    2025-11-06 00:02:19

t2 = conj(phi1);
t3 = conj(phi4);
t4 = cos(phi1);
t5 = cos(phi4);
t6 = sin(phi1);
t7 = sin(phi4);
t8 = cos(t2);
t9 = cos(t3);
t10 = imag(t4);
t11 = real(t4);
t12 = sin(t2);
t13 = sin(t3);
t14 = imag(t6);
t15 = real(t6);
t16 = t4.*(2.1e+1./1.0e+2);
t17 = t5.*(2.1e+1./1.0e+2);
t18 = t4.*(2.1e+1./2.0e+2);
t19 = t5.*(2.1e+1./2.0e+2);
t20 = t6.*(2.1e+1./1.0e+2);
t21 = t7.*(2.1e+1./1.0e+2);
t22 = t6.*(2.1e+1./2.0e+2);
t23 = t7.*(2.1e+1./2.0e+2);
t24 = -t17;
t25 = -t18;
t26 = -t19;
t27 = -t21;
t28 = -t22;
t29 = -t23;
t30 = t8.*(2.1e+1./1.0e+2);
t31 = t9.*(2.1e+1./1.0e+2);
t32 = t8.*(2.1e+1./2.0e+2);
t33 = t9.*(2.1e+1./2.0e+2);
t34 = t10.*(2.1e+1./1.0e+2);
t35 = t11.*(2.1e+1./1.0e+2);
t36 = t12.*(2.1e+1./1.0e+2);
t37 = t13.*(2.1e+1./1.0e+2);
t38 = t12.*(2.1e+1./2.0e+2);
t39 = t13.*(2.1e+1./2.0e+2);
t40 = t14.*(2.1e+1./1.0e+2);
t41 = t15.*(2.1e+1./1.0e+2);
t42 = -t31;
t43 = -t32;
t44 = -t33;
t45 = -t37;
t46 = -t38;
t47 = -t39;
t48 = -t40;
t49 = t16+t24;
t50 = t18+t26;
t51 = t20+t27;
t52 = t22+t29;
t53 = t49.^2;
t54 = t50.^2;
t55 = t51.^2;
t56 = t52.^2;
t57 = t30+t42;
t58 = t32+t44;
t59 = t36+t45;
t60 = t38+t47;
t63 = t6.*t49.*(2.1e+1./5.0e+1);
t64 = t7.*t49.*(2.1e+1./5.0e+1);
t65 = t4.*t51.*(2.1e+1./5.0e+1);
t66 = t5.*t51.*(2.1e+1./5.0e+1);
t73 = t16.*t52;
t75 = t6.*t50.*(-2.1e+1./1.0e+2);
t76 = t7.*t50.*(-2.1e+1./1.0e+2);
t61 = t59.^2;
t62 = t57.^2;
t67 = -t63;
t68 = -t64;
t71 = -t65;
t72 = -t66;
t77 = t12.*t57.*(2.1e+1./5.0e+1);
t78 = t13.*t57.*(2.1e+1./5.0e+1);
t79 = t8.*t59.*(2.1e+1./5.0e+1);
t80 = t9.*t59.*(2.1e+1./5.0e+1);
t87 = t30.*t60;
t89 = t12.*t58.*(-2.1e+1./1.0e+2);
t90 = t13.*t58.*(-2.1e+1./1.0e+2);
t91 = t53+t55;
t81 = -t77;
t82 = -t78;
t85 = -t79;
t86 = -t80;
t92 = t91.^2;
t93 = t61+t62;
t95 = t63+t71;
t96 = t64+t72;
t97 = t19+t25+t91;
t102 = t22+t65+t67;
t103 = t23+t66+t68;
t94 = -t92;
t98 = t77+t85;
t99 = t78+t86;
t100 = 1.0./t97;
t104 = t33+t43+t93;
t107 = t38+t79+t81;
t108 = t39+t80+t82;
t114 = t91.*t95.*2.0;
t115 = t91.*t96.*2.0;
t101 = t100.^2;
t105 = 1.0./t104;
t109 = t54+t56+t94;
t116 = t93.*t98.*2.0;
t117 = t93.*t99.*2.0;
t122 = t73+t75+t114;
t106 = t105.^2;
t110 = sqrt(t109);
t124 = t87+t89+t116;
t111 = conj(t110);
t112 = 1.0./t110;
t118 = t23+t28+t110;
t113 = 1.0./t111;
t119 = t118.^2;
t120 = t39+t46+t111;
t126 = t100.*t118;
t160 = t101.*t102.*t118;
t161 = t101.*t103.*t118;
t162 = (t112.*t122)./2.0;
t163 = (t112.*(t76+t115+t5.*t52.*(2.1e+1./1.0e+2)))./2.0;
t121 = t120.^2;
t127 = atan(t126);
t129 = t101.*t119;
t164 = -t162;
t165 = -t163;
t166 = t106.*t107.*t120;
t167 = t106.*t108.*t120;
t170 = (t113.*t124)./2.0;
t171 = (t113.*(t90+t117+t9.*t60.*(2.1e+1./1.0e+2)))./2.0;
t128 = conj(t127);
t130 = t127.*2.0;
t131 = t129+1.0;
t151 = t106.*t121;
t168 = t18+t164;
t169 = t19+t165;
t172 = -t170;
t173 = -t171;
t132 = t128.*2.0;
t133 = cos(t130);
t134 = sin(t130);
t141 = 1.0./t131;
t152 = t151+1.0;
t174 = t32+t172;
t175 = t33+t173;
t176 = t100.*t168;
t177 = t100.*t169;
t135 = cos(t132);
t136 = imag(t133);
t137 = real(t133);
t138 = sin(t132);
t139 = imag(t134);
t140 = real(t134);
t142 = t133./4.0;
t143 = t134./4.0;
t153 = 1.0./t152;
t178 = t105.*t174;
t179 = t105.*t175;
t190 = t160+t176;
t191 = t161+t177;
t144 = t135./4.0;
t145 = t136./4.0;
t146 = t137./4.0;
t147 = t138./4.0;
t148 = t139./4.0;
t149 = t140./4.0;
t154 = t16+t142;
t155 = t20+t143;
t192 = t166+t178;
t193 = t167+t179;
t196 = t133.*t141.*t190;
t197 = t133.*t141.*t191;
t198 = t134.*t141.*t190;
t199 = t134.*t141.*t191;
t150 = -t148;
t156 = t155.^2;
t157 = t30+t144;
t158 = t36+t147;
t159 = t154.^2;
t180 = t34+t41+t145+t149;
t181 = t180.^2;
t182 = t156+t159;
t183 = t35+t48+t146+t150;
t184 = t183.^2;
t185 = 1.0./t183;
t187 = sqrt(t182);
t186 = 1.0./t184;
t188 = conj(t187);
t194 = t181+t184;
t189 = 1.0./t188;
t195 = 1.0./t194;
T = [(F.*t189.*(t158.*(t30-(t135.*t153.*t192)./2.0).*2.0-t157.*(t36-(t138.*t153.*t192)./2.0).*2.0))./2.0+Tp.*t184.*t195.*(t185.*(t35+t48+imag(t198)./2.0-real(t196)./2.0)+t180.*t186.*(t34+t41-imag(t196)./2.0-real(t198)./2.0));(F.*t189.*(t135.*t153.*t158.*t193-t138.*t153.*t157.*t193))./2.0-Tp.*t184.*t195.*(t185.*(imag(t199)./2.0-real(t197)./2.0)-t180.*t186.*(imag(t197)./2.0+real(t199)./2.0))];
end

== matlab function wbs_sim/controller/locomotion controller/leg length to K ==
  data: L0 input; K output
function K = L2K(L0)
%L2K
%    K = L2K(L0)

%    This function was generated by the Symbolic Math Toolbox version 25.1.
%    2026-01-05 23:54:06

t2 = L0.^2;
t3 = L0.^3;
mt1 = [L0.*(-1.256694061456996e+2)+t2.*2.581523443282094e+2-t3.*2.149318854903044e+2-6.545434024625937];
mt2 = [L0.*(-5.326861058011561e+1)-t2.*1.213324588537186e+2+t3.*2.240124162271842e+2+5.132782040367445e+1];
mt3 = [L0.*(-1.63068095803049e+1)+t2.*2.215867022821785e+1-t3.*1.811887491504631e+1-9.162524414930643e-1];
mt4 = [L0.*(-1.477695717650277e+1)+t2.*1.244339773628746+t3.*1.364406062636162e+1+1.052728646732258e+1];
mt5 = [L0.*(-1.95061975852878e+1)+t2.*4.436685875571423e+1-t3.*3.717617329679582e+1-1.076007147266962];
mt6 = [L0.*(-3.945335551105723e+1)+t2.*4.140049701858666e+1-t3.*1.142809363626002e+1+1.512244887666807e+1];
mt7 = [L0.*(-1.642908725474118e+1)+t2.*3.551097863795313e+1-t3.*2.939807166426749e+1-1.905951578428274];
mt8 = [L0.*(-6.358044102012101e+1)+t2.*1.079663182086489e+2-t3.*7.589855442339257e+1+1.865796046916673e+1];
mt9 = [L0.*(-7.381046954061787e+1)+t2.*7.745323774338758e+1-t3.*2.138000548609193e+1+2.829151127275884e+1];
mt10 = [L0.*3.649275414140703e+2-t2.*8.300279239553372e+2+t3.*6.95502517138432e+2+2.013025045398299e+1];
mt11 = [L0.*(-1.869141318451733e+1)+t2.*2.982522543490013e+1-t3.*1.972612953673563e+1+5.892305887638637];
mt12 = [L0.*7.523484360172975e+1-t2.*1.788813969176453e+2+t3.*1.558805374863315e+2+4.299319245581504e-1];
K = reshape([mt1,mt2,mt3,mt4,mt5,mt6,mt7,mt8,mt9,mt10,mt11,mt12],2,6);
end

== matlab function wbs_sim/controller/right leg transform ==
  data: F input; Tp input; T output; phi1 input; phi4 input
function T = LegTransform(F,Tp,phi1,phi4)
%LegTransform
%    T = LegTransform(F,Tp,PHI1,PHI4)

%    This function was generated by the Symbolic Math Toolbox version 25.1.
%    2025-11-06 00:02:19

t2 = conj(phi1);
t3 = conj(phi4);
t4 = cos(phi1);
t5 = cos(phi4);
t6 = sin(phi1);
t7 = sin(phi4);
t8 = cos(t2);
t9 = cos(t3);
t10 = imag(t4);
t11 = real(t4);
t12 = sin(t2);
t13 = sin(t3);
t14 = imag(t6);
t15 = real(t6);
t16 = t4.*(2.1e+1./1.0e+2);
t17 = t5.*(2.1e+1./1.0e+2);
t18 = t4.*(2.1e+1./2.0e+2);
t19 = t5.*(2.1e+1./2.0e+2);
t20 = t6.*(2.1e+1./1.0e+2);
t21 = t7.*(2.1e+1./1.0e+2);
t22 = t6.*(2.1e+1./2.0e+2);
t23 = t7.*(2.1e+1./2.0e+2);
t24 = -t17;
t25 = -t18;
t26 = -t19;
t27 = -t21;
t28 = -t22;
t29 = -t23;
t30 = t8.*(2.1e+1./1.0e+2);
t31 = t9.*(2.1e+1./1.0e+2);
t32 = t8.*(2.1e+1./2.0e+2);
t33 = t9.*(2.1e+1./2.0e+2);
t34 = t10.*(2.1e+1./1.0e+2);
t35 = t11.*(2.1e+1./1.0e+2);
t36 = t12.*(2.1e+1./1.0e+2);
t37 = t13.*(2.1e+1./1.0e+2);
t38 = t12.*(2.1e+1./2.0e+2);
t39 = t13.*(2.1e+1./2.0e+2);
t40 = t14.*(2.1e+1./1.0e+2);
t41 = t15.*(2.1e+1./1.0e+2);
t42 = -t31;
t43 = -t32;
t44 = -t33;
t45 = -t37;
t46 = -t38;
t47 = -t39;
t48 = -t40;
t49 = t16+t24;
t50 = t18+t26;
t51 = t20+t27;
t52 = t22+t29;
t53 = t49.^2;
t54 = t50.^2;
t55 = t51.^2;
t56 = t52.^2;
t57 = t30+t42;
t58 = t32+t44;
t59 = t36+t45;
t60 = t38+t47;
t63 = t6.*t49.*(2.1e+1./5.0e+1);
t64 = t7.*t49.*(2.1e+1./5.0e+1);
t65 = t4.*t51.*(2.1e+1./5.0e+1);
t66 = t5.*t51.*(2.1e+1./5.0e+1);
t73 = t16.*t52;
t75 = t6.*t50.*(-2.1e+1./1.0e+2);
t76 = t7.*t50.*(-2.1e+1./1.0e+2);
t61 = t59.^2;
t62 = t57.^2;
t67 = -t63;
t68 = -t64;
t71 = -t65;
t72 = -t66;
t77 = t12.*t57.*(2.1e+1./5.0e+1);
t78 = t13.*t57.*(2.1e+1./5.0e+1);
t79 = t8.*t59.*(2.1e+1./5.0e+1);
t80 = t9.*t59.*(2.1e+1./5.0e+1);
t87 = t30.*t60;
t89 = t12.*t58.*(-2.1e+1./1.0e+2);
t90 = t13.*t58.*(-2.1e+1./1.0e+2);
t91 = t53+t55;
t81 = -t77;
t82 = -t78;
t85 = -t79;
t86 = -t80;
t92 = t91.^2;
t93 = t61+t62;
t95 = t63+t71;
t96 = t64+t72;
t97 = t19+t25+t91;
t102 = t22+t65+t67;
t103 = t23+t66+t68;
t94 = -t92;
t98 = t77+t85;
t99 = t78+t86;
t100 = 1.0./t97;
t104 = t33+t43+t93;
t107 = t38+t79+t81;
t108 = t39+t80+t82;
t114 = t91.*t95.*2.0;
t115 = t91.*t96.*2.0;
t101 = t100.^2;
t105 = 1.0./t104;
t109 = t54+t56+t94;
t116 = t93.*t98.*2.0;
t117 = t93.*t99.*2.0;
t122 = t73+t75+t114;
t106 = t105.^2;
t110 = sqrt(t109);
t124 = t87+t89+t116;
t111 = conj(t110);
t112 = 1.0./t110;
t118 = t23+t28+t110;
t113 = 1.0./t111;
t119 = t118.^2;
t120 = t39+t46+t111;
t126 = t100.*t118;
t160 = t101.*t102.*t118;
t161 = t101.*t103.*t118;
t162 = (t112.*t122)./2.0;
t163 = (t112.*(t76+t115+t5.*t52.*(2.1e+1./1.0e+2)))./2.0;
t121 = t120.^2;
t127 = atan(t126);
t129 = t101.*t119;
t164 = -t162;
t165 = -t163;
t166 = t106.*t107.*t120;
t167 = t106.*t108.*t120;
t170 = (t113.*t124)./2.0;
t171 = (t113.*(t90+t117+t9.*t60.*(2.1e+1./1.0e+2)))./2.0;
t128 = conj(t127);
t130 = t127.*2.0;
t131 = t129+1.0;
t151 = t106.*t121;
t168 = t18+t164;
t169 = t19+t165;
t172 = -t170;
t173 = -t171;
t132 = t128.*2.0;
t133 = cos(t130);
t134 = sin(t130);
t141 = 1.0./t131;
t152 = t151+1.0;
t174 = t32+t172;
t175 = t33+t173;
t176 = t100.*t168;
t177 = t100.*t169;
t135 = cos(t132);
t136 = imag(t133);
t137 = real(t133);
t138 = sin(t132);
t139 = imag(t134);
t140 = real(t134);
t142 = t133./4.0;
t143 = t134./4.0;
t153 = 1.0./t152;
t178 = t105.*t174;
t179 = t105.*t175;
t190 = t160+t176;
t191 = t161+t177;
t144 = t135./4.0;
t145 = t136./4.0;
t146 = t137./4.0;
t147 = t138./4.0;
t148 = t139./4.0;
t149 = t140./4.0;
t154 = t16+t142;
t155 = t20+t143;
t192 = t166+t178;
t193 = t167+t179;
t196 = t133.*t141.*t190;
t197 = t133.*t141.*t191;
t198 = t134.*t141.*t190;
t199 = t134.*t141.*t191;
t150 = -t148;
t156 = t155.^2;
t157 = t30+t144;
t158 = t36+t147;
t159 = t154.^2;
t180 = t34+t41+t145+t149;
t181 = t180.^2;
t182 = t156+t159;
t183 = t35+t48+t146+t150;
t184 = t183.^2;
t185 = 1.0./t183;
t187 = sqrt(t182);
t186 = 1.0./t184;
t188 = conj(t187);
t194 = t181+t184;
t189 = 1.0./t188;
t195 = 1.0./t194;
T = [(F.*t189.*(t158.*(t30-(t135.*t153.*t192)./2.0).*2.0-t157.*(t36-(t138.*t153.*t192)./2.0).*2.0))./2.0+Tp.*t184.*t195.*(t185.*(t35+t48+imag(t198)./2.0-real(t196)./2.0)+t180.*t186.*(t34+t41-imag(t196)./2.0-real(t198)./2.0));(F.*t189.*(t135.*t153.*t158.*t193-t138.*t153.*t157.*t193))./2.0-Tp.*t184.*t195.*(t185.*(imag(t199)./2.0-real(t197)./2.0)-t180.*t186.*(imag(t197)./2.0+real(t199)./2.0))];
end

== matlab function wbs_sim/controller/leg controller/left leg feedforward ==
  data: theta input; feedforward output
function feedforward = FFdf(theta)
%FFdf
%    FEEDFORWARD = FFdf(THETA)

%    This function was generated by the Symbolic Math Toolbox version 25.1.
%    2025-12-06 00:25:32

feedforward = (6.37e+2./1.0e+1)./cos(theta);
end
